simulink model "Projeto_Controlador_P"  (R2021a)
settings: Solver=VariableStepAuto  StartTime=0.0  StopTime=10.0  RelTol=1e-3
undefined symbols (not defined in the file or in its folder): H11, id, iq, w
settings Model: Creator=migue  LastModifiedBy=migue

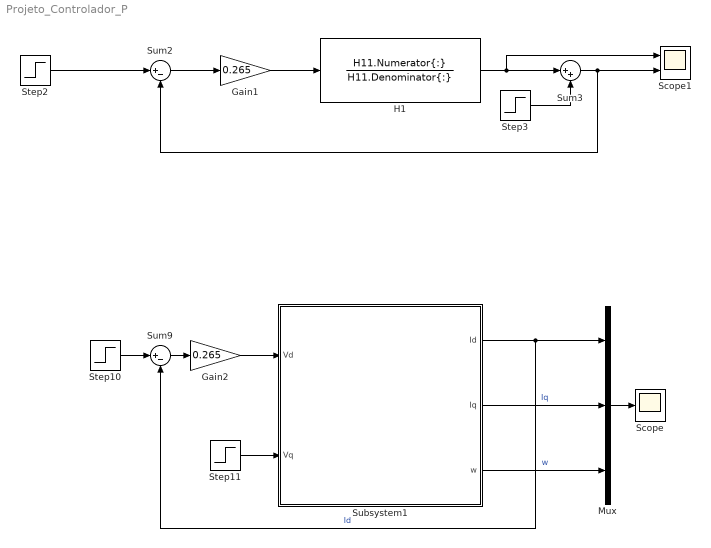
== system Projeto_Controlador_P ==
  Gain1 : Gain  Gain=0.265
  Gain2 : Gain  Gain=0.265
  H1 : TransferFcn  Numerator=H11.Numerator{:}  Denominator=H11.Denominator{:}
  Mux : Mux  Inputs=3
  Scope : Scope
  Scope1 : Scope  NumInputPorts=2
  Step10 : Step  SampleTime=0
  Step11 : Step  Time=1.2  SampleTime=0
  Step2 : Step  SampleTime=0
  Step3 : Step  Time=1.2  SampleTime=0
  Subsystem1 : Subsystem  mask{R=0.16, L=1.3e-4, N=10, J=1.8e-4, b=1e-5, lamb=0.06, Kt=0.095}
      mask prompts: R "Resitência (R)"; L "Indutância(L)"; N "Nº de par de polos(N)"; J "coeficiente(J)"; b "coeficiente(b)"; lamb "(lamb)"; Kt "(Kt)"
  Sum2 : Sum  Inputs=|+-
  Sum3 : Sum  Inputs=|++
  Sum9 : Sum  Inputs=|+-
  wires:
  Sum2/1 -> Gain1/1
  Step3/1 -> Sum3/2
  H1/1 -> Scope1/1, Sum3/1
  Sum3/1 -> Sum2/2, Scope1/2
  Step2/1 -> Sum2/1
  Gain1/1 -> H1/1
  Sum9/1 -> Gain2/1
  Gain2/1 -> Subsystem1/1(Vd)
  Step10/1 -> Sum9/1
  Subsystem1/1(Id) -> Mux/1, Sum9/2  "Id"
  Step11/1 -> Subsystem1/2(Vq)
  Subsystem1/2(Iq) -> Mux/2  "Iq"
  Subsystem1/3(w) -> Mux/3  "w"
  Mux/1 -> Scope/1

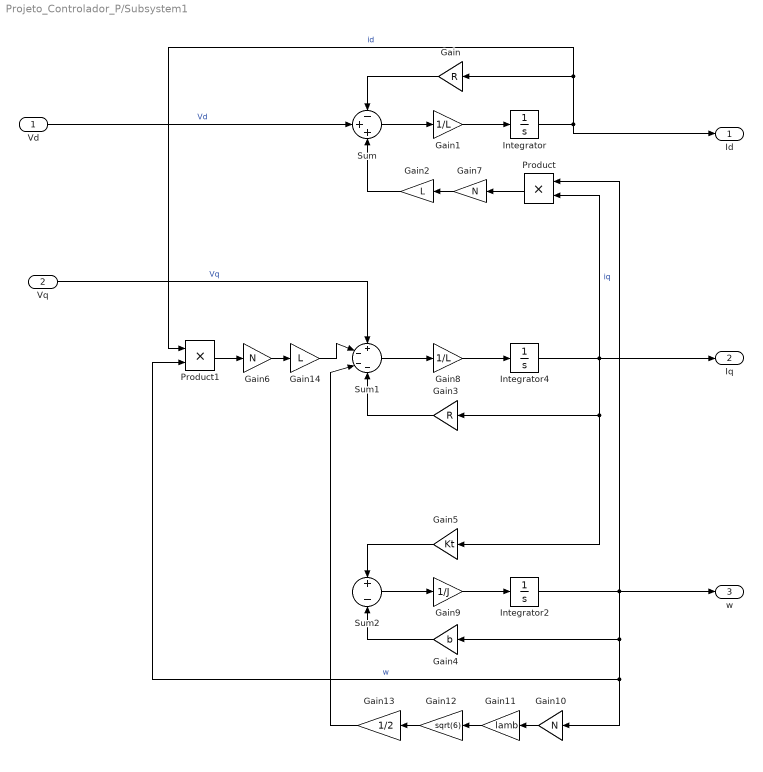
== system Projeto_Controlador_P/Subsystem1 ==
  Vd : Inport
  Vq : Inport  Port=2
  Gain : Gain  Gain=R
  Gain1 : Gain  Gain=1/L
  Gain10 : Gain  Gain=N
  Gain11 : Gain  Gain=lamb
  Gain12 : Gain  Gain=sqrt(6)
  Gain13 : Gain  Gain=1/2
  Gain14 : Gain  Gain=L
  Gain2 : Gain  Gain=L
  Gain3 : Gain  Gain=R
  Gain4 : Gain  Gain=b
  Gain5 : Gain  Gain=Kt
  Gain6 : Gain  Gain=N
  Gain7 : Gain  Gain=N
  Gain8 : Gain  Gain=1/L
  Gain9 : Gain  Gain=1/J
  Integrator : Integrator  InitialCondition=id
  Integrator2 : Integrator  InitialCondition=w
  Integrator4 : Integrator  InitialCondition=iq
  Product : Product
  Product1 : Product
  Sum : Sum  Inputs=-++
  Sum1 : Sum  Inputs=+---
  Sum2 : Sum  Inputs=+-
  Id : Outport
  Iq : Outport  Port=2
  w : Outport  Port=3
  wires:
  Integrator4/1 -> Iq/1, Product/2, Gain3/1, Gain5/1  "iq"
  Integrator/1 -> Gain/1, Product1/1, Id/1  "id"
  Gain8/1 -> Integrator4/1
  Sum1/1 -> Gain8/1
  Product1/1 -> Gain6/1
  Gain/1 -> Sum/1
  Sum2/1 -> Gain9/1
  Integrator2/1 -> w/1, Product/1, Gain10/1, Product1/2, Gain4/1  "w"
  Gain5/1 -> Sum2/1
  Vd/1 -> Sum/2  "Vd"
  Gain9/1 -> Integrator2/1
  Gain1/1 -> Integrator/1
  Sum/1 -> Gain1/1
  Gain4/1 -> Sum2/2
  Gain3/1 -> Sum1/4
  Gain11/1 -> Gain12/1
  Gain10/1 -> Gain11/1
  Product/1 -> Gain7/1
  Vq/1 -> Sum1/1  "Vq"
  Gain12/1 -> Gain13/1
  Gain13/1 -> Sum1/3
  Gain6/1 -> Gain14/1
  Gain7/1 -> Gain2/1
  Gain2/1 -> Sum/3
  Gain14/1 -> Sum1/2
